simulink model "minta2012_jan"  (R2013a)
settings: Solver=ode45  StartTime=0.0  StopTime=3  RelTol=1e-3
values from neighbouring files (symbols this model uses):
  A = zeros(n,m)    [parseLinearSystem.m]    (also in parseSymbolic.m = double(A))
  B = double(B)    [parseSymbolic.m]
undefined symbols (not defined in the file or in its folder): C, D, F, G, H, K, Nu, Nx
settings Model: Creator=rudi  LastModifiedBy=rudi

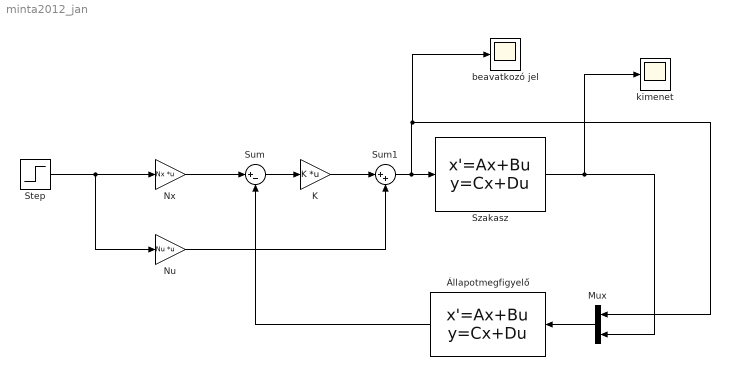
== system minta2012_jan ==
  K : Gain  Gain=K  Multiplication=Matrix(K*u)
  Mux : Mux  Inputs=2
  Nu : Gain  Gain=Nu  Multiplication=Matrix(K*u)
  Nx : Gain  Gain=Nx  Multiplication=Matrix(K*u)
  Step : Step  Time=0  SampleTime=0
  Sum : Sum  Inputs=|+-
  Sum1 : Sum  Inputs=|++
  Szakasz : StateSpace  A=A  B=B  C=C  D=D
  "beavatkozó jel " : Scope
  kimenet : Scope
  Állapotmegfigyelő : StateSpace  A=F  B=[H,G]  C=eye(4)  D=zeros(4,2)
  wires:
  Mux/1 -> Állapotmegfigyelő/1
  Szakasz/1 -> kimenet/1, Mux/2
  Sum/1 -> K/1
  Állapotmegfigyelő/1 -> Sum/2
  K/1 -> Sum1/1
  Nu/1 -> Sum1/2
  Sum1/1 -> "beavatkozó jel "/1, Mux/1, Szakasz/1
  Nx/1 -> Sum/1
  Step/1 -> Nu/1, Nx/1
